simulink library "DQN_Lib (conflicted copy 2023-11-25 155310)"  (R2023b)
settings: Solver=VariableStepAuto  StartTime=0.0  StopTime=10.0  RelTol=1e-3
undefined symbols (not defined in the file): FreqRad, HrmOrd, Init, La, N, R, Ra, TimeStep, Ts, Ts_dqn, Ws
libraries: $bdroot x4, spsMeanVariableFrequencyLib x4, eeTransforms x3, spsabctodq0Lib x2, spsAlphaBetaZerotodq0Lib x1
(part 6 of 8)

== matlab function DQN_Lib (conflicted copy 2023-11-25 155310)/BACKUP/Int_DQNc_Mat1 ==
  settings: updateMethod=DISCRETE
  data: Xpnz input; N parameter; dt parameter; w parameter; InitInt parameter; Zpnz output; R parameter; iL parameter; swFeed parameter
function Zpnz    = Int_DQN_Mat(Xpnz, N, dt, w, InitInt, R, iL, swFeed)

    nrSig = 1;

    Zpnz = complex(zeros(3,N+1));

    persistent Zpnz_old;
    persistent Xpnz_old;
    persistent Krl1;
    persistent Krl2;
    persistent dt2;

        
        
    if(isempty(Zpnz_old)) 
    
        a = -0.5+0.866i;
        a2 = -0.5-0.866i;
        Sas = [1,a,a2;1,a2,a;1,1,1]/3;
        
        Zpnz_old = complex(zeros(3,N+1));
        Xpnz_old = complex(zeros(3,N+1));
        
        if(~isempty(InitInt))
        Zpnz_old(:,1) = Sas * InitInt;
        
        end
        dt2 = dt/2;

        if(swFeed)
            Krl1 = (iL/(1+dt2*R*iL));
            Krl2 = (1-dt2*R*iL)/(1+dt2*R*iL);
        else
            Krl1 = 1;
            Krl2 = 1;
        end
            
    end
       
    
    for k = 1 : nrSig
    
        %Zpnz(:,1) = dt2*(Xpnz(:,1)+Xpnz_old(:,1)) + Zpnz_old(:,1);

        Zpnz(:,1) = Krl1*dt2*(Xpnz(:,1)+Xpnz_old(:,1))+Krl2*Zpnz_old(:,1);

        Xpnz_old(:,1) = Xpnz(:,1);
        Zpnz_old(:,1) = Zpnz(:,1);


        if(N>0)

            for i = 1 : N
                wn =  i * w; 
                wndt2 = wn*dt2;

                A = 2*dt2/(1+wndt2^2);
                B = (1-wndt2^2)/(1+wndt2^2);

                % Zdp(i) = Krl1*A*(real(Xpnz(1,i+1))+wndt2*imag(Xpnz(1,i+1)))+Krl2*(B*real(Zpnz(1,i+1))+A*wn*imag(Zpnz(1,i+1)));
                % Zqp(i) = Krl1*A*(imag(Xpnz(1,i+1))-wndt2*real(Xpnz(1,i+1)))+Krl2*(B*imag(Zpnz(1,i+1))-A*wn*real(Zpnz(1,i+1)));

                %%% POS %%%
                Zpnz(1,i+1) =     Krl1*A*(real(Xpnz(1,i+1))+wndt2*imag(Xpnz(1,i+1)))+Krl2*(B*real(Zpnz_old(1,i+1))+A*wn*imag(Zpnz_old(1,i+1))) ...
                            + 1i*(Krl1*A*(imag(Xpnz(1,i+1))-wndt2*real(Xpnz(1,i+1)))+Krl2*(B*imag(Zpnz_old(1,i+1))-A*wn*real(Zpnz_old(1,i+1))));

                %%% NEG %%%
                Zpnz(2,i+1) =     Krl1*A*(real(Xpnz(2,i+1))+wndt2*imag(Xpnz(2,i+1)))+Krl2*(B*real(Zpnz_old(2,i+1))+A*wn*imag(Zpnz_old(2,i+1))) ...
                            + 1i*(Krl1*A*(imag(Xpnz(2,i+1))-wndt2*real(Xpnz(2,i+1)))+Krl2*(B*imag(Zpnz_old(2,i+1))-A*wn*real(Zpnz_old(2,i+1))));

                %%% ZERO %%%
                Zpnz(3,i+1) =     Krl1*A*(real(Xpnz(3,i+1))+wndt2*imag(Xpnz(3,i+1)))+Krl2*(B*real(Zpnz_old(3,i+1))+A*wn*imag(Zpnz_old(3,i+1))) ...
                            + 1i*(Krl1*A*(imag(Xpnz(3,i+1))-wndt2*real(Xpnz(3,i+1)))+Krl2*(B*imag(Zpnz_old(3,i+1))-A*wn*real(Zpnz_old(3,i+1))));


                Zpnz_old(:,i+1) = Zpnz(:,i+1);


            end

        end

    end
end
